simulink model "P_decouple_cascade_rov"  (Simulink 6.0)
settings: Solver=ode45  StartTime=0.0  StopTime=650  RelTol=1e-3
undefined symbols (not defined in the file): B, DQ, DQL, I, m, M, Ma, MaL, MaU, rg, sigbuilder_block, T, W, xb, xg, Xudot, yb, yg, Yvdot, zb, zg, Zwdot
libraries: simulink_extras x27, simulink x20
(part 1 of 5)
settings Model: LastModifiedBy=c chin

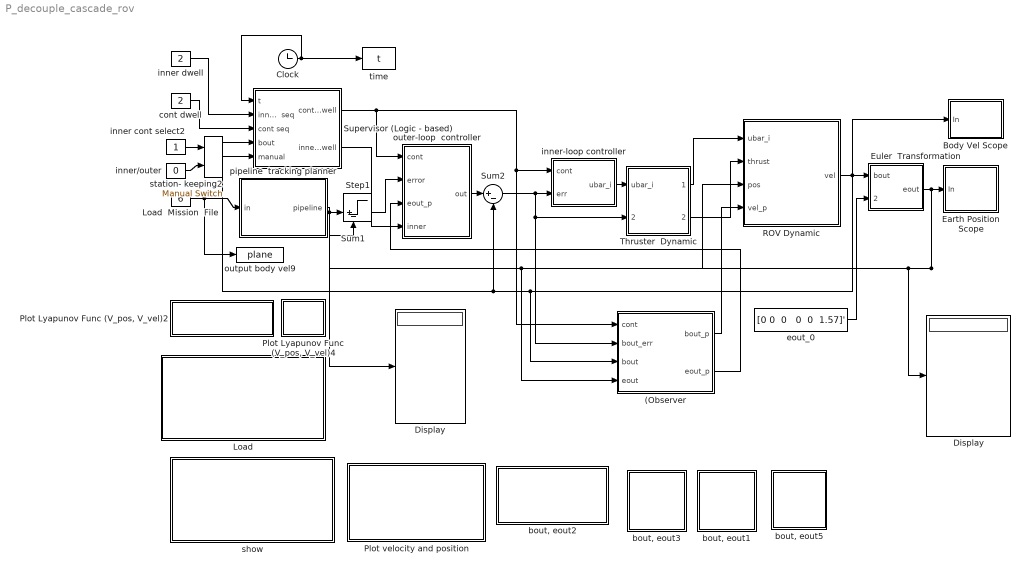
== system P_decouple_cascade_rov ==
  " Load  " : Subsystem  AncestorBlock=|
      | rov_design_analysis/ROV Controller
      | Design
      | Applications/ Load RRCROV2 parameters
      settings: OpenFcn=|
      | clc
      | cd c:\Matlab7\toolbox\rov_design_analysis\\mat_file ;
      | load rrcrovf;
      mask Display: disp('Double-click \n to \n Load the\n RRCROV\n parameters')
  " ROV Dynamic   " : Subsystem
      mask Display:
      | disp('ROV')
      | image(imread('/rov_design_analysis/fig/ROVRRC2.jpg'));
      | color('white');port_label('input',1,'ubar_i')
      | color('white');port_label('input',2,'thrust')
      | color('white');port_label('input',3,'MCD_select')
      | color('white');port_label('input',4,'eout')
      | color('white');port_label('input',5,'bout_p')
      | 
      | color('white');port_label('output',1,'vel')
      | color('white');port_label('output',2,'boutdot')
  " inner dwell" : Constant  Value=2
  " station- keeping2" : simulink/Signal Routing/Manual Switch  sw=1  action=0
  (Observer : Subsystem
      mask Display: disp('Observer')
  Body Vel Scope : Subsystem  AncestorBlock=|
      | rov_design_analysis/ROV Controller
      | Design
      | Applications/1. Heading autopilot/Earth Position
      | Scope
      mask Display: disp('Body\nVelocity\nScope')
  Clock : Clock
      settings: Decimation=10
  Display : Display
  "Display " : Display
  "Earth Position Scope " : Subsystem  AncestorBlock=|
      | rov_design_analysis/ROV Controller
      | Design
      | Applications/1. Heading autopilot/Earth Position
      | Scope
      mask Display: disp('Earth\nPosition\nScope')
  Euler  Transformation : Subsystem  AncestorBlock=rov_design_analysis/Scope Utilities/Euler Transformation
      mask Display: disp('Navigation \n Sensor')
  Load  Mission  File : Constant  Value=6
  "Plot Lyapunov Func (V_pos, V_vel)2" : Subsystem  AncestorBlock=|
      | rov_design_analysis/ROV Controller
      | Design
      | Applications/Plot velocity and position
      settings: OpenFcn=|
      | clc
      | close all
      mask Display: disp('Close All Figure')
  "Plot Lyapunov Func (V_pos, V_vel)4" : Subsystem  AncestorBlock=|
      | rov_design_analysis/ROV Controller
      | Design
      | Applications/Plot velocity and position
      settings: OpenFcn=|
      | clc
      | clear
      mask Display: disp('Clear')
  Plot velocity and position : Subsystem  AncestorBlock=|
      | rov_design_analysis/ROV Controller
      | Design
      | Applications/Plot velocity and position
      settings: OpenFcn=|
      | clc
      | cd c:\Matlab7\toolbox\rov_design_analysis\\m_file ;
      | run nonlin_resp6
      mask Display: disp('Double-click \n to \n Plot Velocity \n and \n Position')
  Sum1 : Sum  Inputs=|+-  OutDataTypeMode=double  SaturateOnIntegerOverflow=on
  Sum2 : Sum  Inputs=|+-  OutDataTypeMode=double  SaturateOnIntegerOverflow=on
  Supervisor (Logic - based) : Subsystem
      mask Display: disp('Supervisor \n (Logic-based)')
  Thruster  Dynamic : Subsystem
      mask Display: disp('Thruster \n Dynamic')
  "bout, eout1" : Subsystem  AncestorBlock=|
      | rov_design_analysis/ROV Controller
      | Design
      | Applications/Plot velocity and position
      settings: OpenFcn=|
      | clc
      | cd c:\Matlab7\toolbox\rov_design_analysis\\m_file ;
      | figure
      | plot(eout(:,1),-eout(:,3))
      | xlabel('x')
      | ylabel('z')
      mask Display: disp('Plot \n XZ ')
  "bout, eout2" : Subsystem  AncestorBlock=|
      | rov_design_analysis/ROV Controller
      | Design
      | Applications/Plot velocity and position
      settings: OpenFcn=|
      | clc
      | cd c:\Matlab7\toolbox\rov_design_analysis\\m_file ;
      | figure
      | plot3(eout(:,1), eout(:,2),-eout(:,3))
      | xlabel('x')
      | ylabel('y')
      | zlabel('z')
      | grid on
      mask Display: disp('Plot \n 3D Response')
  "bout, eout3" : Subsystem  AncestorBlock=|
      | rov_design_analysis/ROV Controller
      | Design
      | Applications/Plot velocity and position
      settings: OpenFcn=|
      | clc
      | cd c:\Matlab7\toolbox\rov_design_analysis\\m_file ;
      | figure
      | plot(eout(:,1), eout(:,2))
      | xlabel('x')
      | ylabel('y')
      mask Display: disp('Plot \n XY ')
  "bout, eout5" : Subsystem  AncestorBlock=|
      | rov_design_analysis/ROV Controller
      | Design
      | Applications/Plot velocity and position
      settings: OpenFcn=|
      | clc
      | cd c:\Matlab7\toolbox\rov_design_analysis\\m_file ;
      | figure
      | box off
      | subplot(4,1,1)
      | plot(inner.time,inner.signals.values)
      | xlabel('time (sec)')
      | ylabel('Inner controller type')
      | subplot(4,1,2)
      | plot(outer.time,outer.signals.values)
      | xlabel('time (sec)')
      | ylabel('Outer controller type')
      | subplot(4,1,3)
      | plot(plane.time,plane.signals.values)
      | xlabel('time (sec)')
      | ylabel('Input sequence')
      | 
      | subplot(4,1,4)
      | plot(inner_only.time,inner_only.signals.values)
      | xlabel('time (sec)')
      | ylabel('Inner/Outer loop')
      mask Display: disp('Plot \n switching \n signal ')
  cont dwell : Constant  Value=2
  eout_0 : Constant  Value="[0 0  0   0  0  1.57]'"  OutDataTypeMode=double
  inner cont select2 : Constant
  inner-loop controller : Subsystem  Description=f(x)  AncestorBlock=|
      | rov_design_analysis/ROV Controller
      | Design
      | Applications/1. Heading autopilot/controller
      mask Display: disp('Inner Loop \n Controller')
  "inner/outer  " : Constant  Value=0
  outer-loop  controller : Subsystem  Description=f(x)  AncestorBlock=|
      | rov_design_analysis/ROV Controller
      | Design
      | Applications/1. Heading autopilot/controller
      mask Display: disp('Outer Loop \n Controller')
  output body vel9 : ToWorkspace  VariableName=plane  SampleTime=1  SaveFormat=Structure With Time
  "pipeline  tracking planner  " : Subsystem  AncestorBlock=|
      | rov_design_analysis/ROV Controller
      | Design
      | Applications/1. Heading autopilot/pipe tracking
      | profile
      | (Auto)
      mask Display: disp('Pipeline Tracking \n Planner')
  show : Subsystem  AncestorBlock=|
      | rov_design_analysis/ROV Controller
      | Design
      | Applications/ Load RRCROV2 parameters
      settings: OpenFcn=|
      | clc
      | cd  c:\Matlab7\toolbox\rov_design_analysis\hybrid ;
      | open rrcrov2_para
      mask Display: disp('Double-click \n to \n SHOW\n RRCROV\n parameters')
  time : ToWorkspace  VariableName=t  SampleTime=1  SaveFormat=Array
  Step1 : Step  IOType=siggen  SampleTime=0
  wires:
  " ROV Dynamic   "/1(vel) -> Euler  Transformation/1(bout), (Observer/3(bout), Sum2/2, Supervisor (Logic - based)/4(bout), Body Vel Scope/1(In)
  Euler  Transformation/1(eout) -> "Earth Position Scope "/1(In), (Observer/4(eout), Sum1/2, " ROV Dynamic   "/3("pos "), "Display "/1
  Clock/1 -> time/1, Supervisor (Logic - based)/1(t)
  Thruster  Dynamic/2(thruster_out) -> " ROV Dynamic   "/2("thrust ")
  Sum2/1 -> Thruster  Dynamic/2(bout_err), (Observer/2(bout_err), inner-loop controller/2(err)
  Thruster  Dynamic/1(cont_out) -> " ROV Dynamic   "/1(ubar_i)
  inner-loop controller/1(ubar_i) -> Thruster  Dynamic/1(ubar_i)
  (Observer/2(eout_p) -> outer-loop  controller/3(eout_p)
  (Observer/1(bout_p) -> " ROV Dynamic   "/4(vel_p)
  "pipeline  tracking planner  "/1(pipeline) -> Sum1/1, Display/1
  Supervisor (Logic - based)/1(cont dwell) -> inner-loop controller/1(cont), (Observer/1(cont), outer-loop  controller/1(cont)
  outer-loop  controller/1(out) -> Sum2/1
  Supervisor (Logic - based)/2(inner  dwell) -> outer-loop  controller/4(inner)
  " inner dwell"/1 -> Supervisor (Logic - based)/2(inner  seq)
  cont dwell/1 -> Supervisor (Logic - based)/3(cont seq)
  eout_0/1 -> Euler  Transformation/2(eout_0)
  Load  Mission  File/1 -> output body vel9/1, "pipeline  tracking planner  "/1(in)
  inner cont select2/1 -> " station- keeping2"/1
  "inner/outer  "/1 -> " station- keeping2"/2
  " station- keeping2"/1 -> Supervisor (Logic - based)/5(manual)
  Sum1/1 -> outer-loop  controller/2(error)

== system P_decouple_cascade_rov/ Load   ==

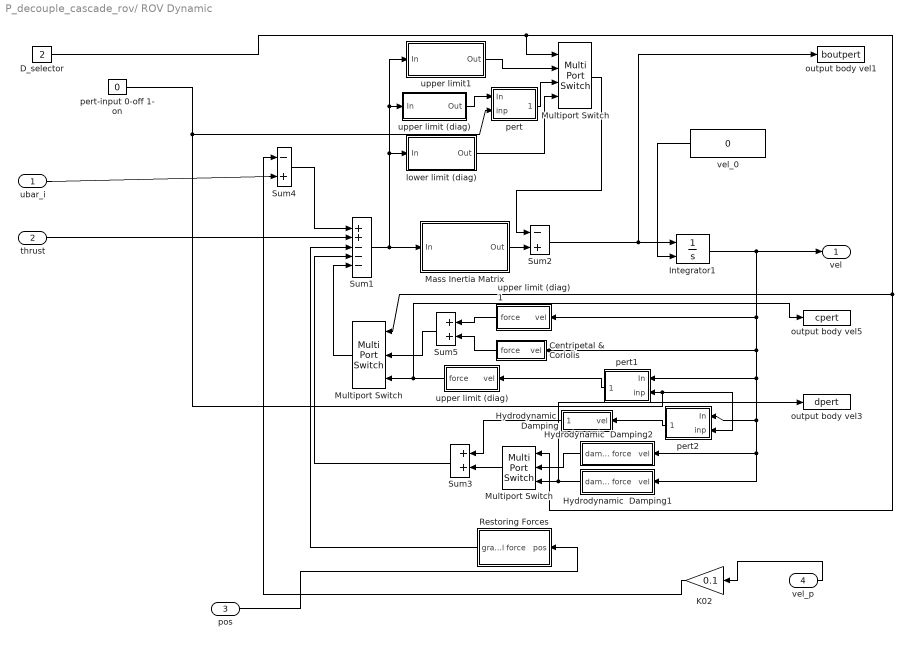
== system P_decouple_cascade_rov/ ROV Dynamic    ==
  ubar_i : Inport  Port=1  LatchInput=off
  "thrust " : Inport  Port=2  LatchInput=off
  "pos " : Inport  Port=3  LatchInput=off
  vel_p : Inport  Port=4  LatchInput=off
  Centripetal & Coriolis : Subsystem  Orientation=left  AncestorBlock=rov_design_analysis/ROV Models/1. Six DOF RRC ROV II/Centripetal & Coriolis
      mask Display: disp('C')
  D_selector : Constant  Value=2
  Hydrodynamic  Damping : Subsystem  Orientation=left
      mask Display: disp('D')
  Hydrodynamic  Damping1 : Subsystem  Orientation=left
      mask Display: disp('perturb \nDamping')
  Hydrodynamic  Damping2 : Subsystem  Orientation=left
      mask Display: disp('Zero Perturb')
  Integrator1 : Integrator  InitialConditionSource=external
  K02 : Gain  Orientation=left  Gain=0.1  SaturateOnIntegerOverflow=on
  Mass Inertia Matrix : Subsystem
      mask Display: disp('inv(MRB+MA)')
  Multiport Switch : MultiPortSwitch  Inputs=3
  "Multiport Switch  " : MultiPortSwitch  Orientation=left  Inputs=2
  "Multiport Switch    " : MultiPortSwitch  Orientation=left  Inputs=2
  Restoring Forces : Subsystem  Orientation=left
      mask Display: disp('Restoring\nForce')
  Sum1 : Sum  Inputs=++---  SaturateOnIntegerOverflow=on  InputSameDT=on
  Sum2 : Sum  Inputs=-+  SaturateOnIntegerOverflow=on  InputSameDT=on
  Sum3 : Sum  Orientation=left  SaturateOnIntegerOverflow=on  InputSameDT=on
  Sum4 : Sum  Inputs=|-+  SaturateOnIntegerOverflow=on  InputSameDT=on
  Sum5 : Sum  Orientation=left  SaturateOnIntegerOverflow=on  InputSameDT=on
  lower limit (diag) : Subsystem
      mask Display: disp('Perturb MA')
  output body vel1 : ToWorkspace  VariableName=boutpert  SampleTime=1  SaveFormat=Array
  output body vel3 : ToWorkspace  VariableName=dpert  SampleTime=1  SaveFormat=Array
  output body vel5 : ToWorkspace  VariableName=cpert  SampleTime=1  SaveFormat=Array
  pert : Subsystem
  pert-input 0-off 1- on : Constant  Value=0
  pert1 : Subsystem  Orientation=left
  pert2 : Subsystem  Orientation=left
  upper limit (diag) : Subsystem
      mask Display: disp('Perturb MA')
  "upper limit (diag)   " : Subsystem  Orientation=left
      mask Display: disp('Perturb CA')
  upper limit (diag)   1 : Subsystem  Orientation=left
      mask Display: disp('CA')
  upper limit1 : Subsystem
      mask Display: disp('Zero Perturb')
  vel_0 : Constant  Orientation=left  Value=0  OutDataTypeMode=double
  vel : Outport
  wires:
  Restoring Forces/1(gravitational force) -> Sum1/3
  "thrust "/1 -> Sum1/2
  Sum1/1 -> Mass Inertia Matrix/1(In), upper limit1/1(In), upper limit (diag)/1(In), lower limit (diag)/1(In)
  "Multiport Switch  "/1 -> Sum1/5
  "pos "/1 -> Restoring Forces/1(pos)
  Mass Inertia Matrix/1(Out) -> Sum2/2
  upper limit1/1(Out) -> Multiport Switch/2
  lower limit (diag)/1(Out) -> Multiport Switch/4
  Multiport Switch/1 -> Sum2/1
  "upper limit (diag)   "/1(force) -> "Multiport Switch  "/3, output body vel5/1
  Sum5/1 -> "Multiport Switch  "/2
  Hydrodynamic  Damping1/1(damping force) -> "Multiport Switch    "/3, output body vel3/1
  Hydrodynamic  Damping2/1(damping force) -> "Multiport Switch    "/2
  Sum3/1 -> Sum1/4
  "Multiport Switch    "/1 -> Sum3/2
  Hydrodynamic  Damping/1(damping force) -> Sum3/1
  upper limit (diag)   1/1(force) -> Sum5/1
  Centripetal & Coriolis/1(force) -> Sum5/2
  Sum2/1 -> output body vel1/1, Integrator1/1
  Integrator1/1 -> vel/1, upper limit (diag)   1/1(vel), Centripetal & Coriolis/1(vel), Hydrodynamic  Damping1/1(vel), Hydrodynamic  Damping2/1(vel), pert2/1(In), pert1/1(In)
  vel_0/1 -> Integrator1/2
  K02/1 -> Sum4/1
  ubar_i/1 -> Sum4/2
  Sum4/1 -> Sum1/1
  vel_p/1 -> K02/1
  pert2/1(on/off) -> Hydrodynamic  Damping/1(vel)
  pert1/1(on/off) -> "upper limit (diag)   "/1(vel)
  upper limit (diag)/1(Out) -> pert/1(In)
  pert/1(on/off) -> Multiport Switch/3
  pert-input 0-off 1- on/1 -> pert/2(inp), pert1/2(inp), pert2/2(inp)
  D_selector/1 -> Multiport Switch/1, "Multiport Switch  "/1, "Multiport Switch    "/1

== system P_decouple_cascade_rov/(Observer ==
  cont : Inport  Port=1  LatchInput=off
  bout_err : Inport  Port=2  LatchInput=off
  bout : Inport  Port=3  LatchInput=off
  eout : Inport  Port=4  LatchInput=off
  " Six DOF RRC ROV   1" : Subsystem
      mask Display:
      | disp('ROV')
      | image(imread('/rov_design_analysis/fig/ROVRRC2.jpg'));
      | color('white');port_label('input',1,'ubar_i')
      | color('white');port_label('input',2,'thrust')
      | color('white');port_label('input',3,'MCD_select')
      | color('white');port_label('input',4,'pos')
      | color('white');port_label('output',1,'vel')
      | color('white');port_label('output',2,'Inv_MC')
  Euler  Transformation1 : Subsystem  AncestorBlock=rov_design_analysis/Scope Utilities/Euler Transformation
  MCD_selector : Constant  Value=2
  Sum1 : Sum  Inputs=-+  SaturateOnIntegerOverflow=on  InputSameDT=on
  Sum2 : Sum  Inputs=-+  SaturateOnIntegerOverflow=on  InputSameDT=on
  Thruster  Dynamic : Subsystem
  eout_hat_0 : Constant  Orientation=left  Value=0  OutDataTypeMode=double
  inner-loop controller1 : Subsystem  Description=f(x)  AncestorBlock=|
      | rov_design_analysis/ROV Controller
      | Design
      | Applications/1. Heading autopilot/controller
  output body vel2 : ToWorkspace  VariableName=boutupert  SampleTime=1  SaveFormat=Array
  output body vel4 : ToWorkspace  VariableName=eoutupert  SampleTime=1  SaveFormat=Array
  bout_p : Outport
  eout_p : Outport  Port=2
  wires:
  " Six DOF RRC ROV   1"/1(vel) -> Euler  Transformation1/1(vel), Sum2/1, output body vel2/1
  MCD_selector/1 -> " Six DOF RRC ROV   1"/3(MCD_select), inner-loop controller1/3(M_select)
  bout_err/1 -> Thruster  Dynamic/2(bout_err), inner-loop controller1/2(err)
  Euler  Transformation1/1(eout_hat) -> " Six DOF RRC ROV   1"/4("pos "), Sum1/1, output body vel4/1
  eout_hat_0/1 -> Euler  Transformation1/2(eta_0)
  bout/1 -> Sum2/2
  eout/1 -> Sum1/2
  Sum2/1 -> bout_p/1
  Sum1/1 -> eout_p/1
  Thruster  Dynamic/1(cont_out) -> " Six DOF RRC ROV   1"/1(ubar_i)
  inner-loop controller1/1(ubar_i) -> Thruster  Dynamic/1(ubar_i)
  Thruster  Dynamic/2(thruster_out) -> " Six DOF RRC ROV   1"/2("thrust ")
  cont/1 -> inner-loop controller1/1(cont)

== system P_decouple_cascade_rov/Body Vel Scope ==
  In : Inport  Port=1  LatchInput=off
  Demux : Demux  Outputs=6
  output body vel4 : ToWorkspace  VariableName=bout  SampleTime=1  SaveFormat=Array
  phi : Scope
      settings: TickLabels=on  YMin=-0.125  YMax=0.2  DataFormat=Array
  theta : Scope
      settings: TickLabels=on  TimeRange=200  YMin=-0.05  YMax=0.15  DataFormat=Array
  x : Scope
      settings: TickLabels=on  TimeRange=50  YMin=-0.025  YMax=0.375  DataFormat=Array
  y : Scope
      settings: TickLabels=on  YMin=-0.02  YMax=0.1  DataFormat=Array
  yaw : Scope
      settings: TickLabels=on  TimeRange=200  YMin=-0.05  YMax=0.15  SaveName=ScopeData2  DataFormat=Array
  z : Scope
      settings: TickLabels=on  TimeRange=50  YMin=-0.0025  YMax=0.0375  DataFormat=Array
  wires:
  Demux/5 -> theta/1
  In/1 -> Demux/1, output body vel4/1
  Demux/3 -> z/1
  Demux/4 -> phi/1
  Demux/2 -> y/1
  Demux/1 -> x/1
  Demux/6 -> yaw/1

== system P_decouple_cascade_rov/Earth Position Scope  ==
  In : Inport  Port=1  LatchInput=off
  Demux : Demux  Outputs=6
  XY Graph : simulink/Sinks/XY Graph  xmin=-50  xmax=50  ymin=-50  ymax=50  st=-1
  output body vel5 : ToWorkspace  VariableName=eout  SampleTime=1  SaveFormat=Array
  phi : Scope
      settings: TickLabels=on  YMin=-0.125  YMax=0.2  DataFormat=Array
  theta : Scope
      settings: TickLabels=on  TimeRange=200  YMin=-0.05  YMax=0.15  DataFormat=Array
  x : Scope
      settings: TickLabels=on  TimeRange=50  YMin=-0.025  YMax=0.375  DataFormat=Array
  y : Scope
      settings: TickLabels=on  YMin=-0.02  YMax=0.1  DataFormat=Array
  yaw : Scope
      settings: TickLabels=on  TimeRange=200  YMin=-0.05  YMax=0.15  SaveName=ScopeData2  DataFormat=Array
  z : Scope
      settings: TickLabels=on  TimeRange=50  YMin=-0.0025  YMax=0.0375  DataFormat=Array
  wires:
  Demux/5 -> theta/1
  In/1 -> Demux/1, output body vel5/1
  Demux/3 -> z/1
  Demux/4 -> phi/1
  Demux/2 -> y/1, XY Graph/2
  Demux/1 -> x/1, XY Graph/1
  Demux/6 -> yaw/1

== system P_decouple_cascade_rov/Euler  Transformation ==
  bout : Inport  Port=1  LatchInput=off
  eout_0 : Inport  Port=2  LatchInput=off
  Demux : Demux  Outputs=2
  Demux1 : Demux  Outputs=2
  Intregrator2 : Integrator  InitialConditionSource=external
  Mux1 : Mux  Inputs=2
  Terminator : Terminator
  Transformation matrix R : Subsystem
      mask Display: disp('Transformation R')
  Transformation matrix T : Subsystem
      mask Display: disp('Transformation T')
  output body vel1 : ToWorkspace  VariableName=eoutpert  SampleTime=1  SaveFormat=Array
  eout : Outport  InitialOutput=0
  wires:
  Mux1/1 -> Intregrator2/1
  Intregrator2/1 -> Demux1/1, eout/1, output body vel1/1
  Demux/2 -> Transformation matrix R/1(angular body  velocity)
  Demux/1 -> Transformation matrix T/1(translational body velocity)
  bout/1 -> Demux/1
  Demux1/2 -> Transformation matrix T/2(angular position), Transformation matrix R/2(angular position)
  Transformation matrix R/1(angular earth velocity) -> Mux1/2
  Transformation matrix T/1(translational earth velocity) -> Mux1/1
  Demux1/1 -> Terminator/1
  eout_0/1 -> Intregrator2/2

== system P_decouple_cascade_rov/Plot Lyapunov Func (V_pos, V_vel)2 ==

== system P_decouple_cascade_rov/Plot Lyapunov Func (V_pos, V_vel)4 ==

== system P_decouple_cascade_rov/Plot velocity and position ==

== system P_decouple_cascade_rov/Supervisor (Logic - based) ==
  t : Inport  Port=1  LatchInput=off
  inner  seq : Inport  Port=2  LatchInput=off
  cont seq : Inport  Port=3  LatchInput=off
  bout : Inport  Port=4  LatchInput=off
  manual : Inport  Port=5  LatchInput=off
  150-300 : Relay  OnSwitchValue=150  OffSwitchValue=0  OnOutputValue=0  OffOutputValue=1
  Constant1 : Constant
  Constant8 : Constant
  Gain : Gain  Gain=0.5
  Mass Inertia Matrix1 : Subsystem
      mask Display: disp('MRB+MA')
  Math Function1 : Math  Operator=square  SaturateOnIntegerOverflow=on
  Subsystem : Subsystem
  Switching sequence : Subsystem  AncestorBlock=rov_design_analysis/Scope Utilities/Switching sequence
      mask Display: disp('Dwell \n Sequence')
  Switching sequence1 : Subsystem  AncestorBlock=rov_design_analysis/Scope Utilities/Switching sequence
      mask Display: disp('Dwell \n Sequence')
  "cont dwell switch  " : MultiPortSwitch  Inputs=2
  inner dwell Switch : MultiPortSwitch  Inputs=3
  output body vel6 : ToWorkspace  VariableName=outer  SampleTime=1  SaveFormat=Structure With Time
  output body vel8 : ToWorkspace  VariableName=inner_only  SampleTime=1  SaveFormat=Structure With Time
  cont dwell : Outport
  inner  dwell : Outport  Port=2
  wires:
  inner  seq/1 -> inner dwell Switch/1
  150-300/1 -> inner dwell Switch/2  "1"
  Constant8/1 -> inner dwell Switch/3  "2"
  inner dwell Switch/1 -> Subsystem/1(In)
  cont seq/1 -> "cont dwell switch  "/1
  "cont dwell switch  "/1 -> cont dwell/1, output body vel6/1
  t/1 -> 150-300/1
  Switching sequence1/1(" ") -> "cont dwell switch  "/2
  Constant1/1 -> "cont dwell switch  "/3
  Switching sequence/1(" ") -> inner dwell Switch/4  "3"
  Subsystem/1(inner dwell) -> inner  dwell/1, output body vel8/1
  manual/1 -> Subsystem/3(manual)
  bout/1 -> Math Function1/1
  Math Function1/1 -> Mass Inertia Matrix1/1(In)
  Mass Inertia Matrix1/1(Out) -> Gain/1
  Gain/1 -> Subsystem/2(V)

== system P_decouple_cascade_rov/Thruster  Dynamic ==
  ubar_i : Inport  Port=1  LatchInput=off
  bout_err : Inport  Port=2  LatchInput=off
  Sum2 : Sum  Inputs=|++  OutDataTypeMode=double  SaturateOnIntegerOverflow=on
  Thruster configuration1 : Subsystem  AncestorBlock=|
      | rov_design_analysis/ROV Controller
      | Design
      | Applications/1. Heading autopilot/Thruster
      | configuration
      mask Display: disp('T')
  Thruster configuration4 : Subsystem  AncestorBlock=|
      | rov_design_analysis/ROV Controller
      | Design
      | Applications/1. Heading autopilot/Thruster
      | configuration
      mask Display: disp('T')
  output earth pos1 : ToWorkspace  VariableName=thrustdc  SampleTime=1  SaveFormat=Array
  output earth pos2 : ToWorkspace  VariableName=thrustd  SampleTime=1  SaveFormat=Array
  output earth pos3 : ToWorkspace  VariableName=thrust  SampleTime=1  SaveFormat=Array
  thruster  dynamic     1 : Subsystem
  cont_out : Outport
  thruster_out : Outport  Port=2
  wires:
  Thruster configuration1/1(output force) -> thruster_out/1
  Thruster configuration4/1(output force) -> cont_out/1
  thruster  dynamic     1/1(T) -> Thruster configuration1/1(input velocity), Sum2/2, output earth pos3/1
  bout_err/1 -> thruster  dynamic     1/1(volt)
  ubar_i/1 -> Thruster configuration4/1(input velocity), Sum2/1, output earth pos1/1
  Sum2/1 -> output earth pos2/1

== system P_decouple_cascade_rov/bout, eout1 ==

== system P_decouple_cascade_rov/bout, eout2 ==

== system P_decouple_cascade_rov/bout, eout3 ==

== system P_decouple_cascade_rov/bout, eout5 ==

== system P_decouple_cascade_rov/inner-loop controller ==
  cont : Inport  Port=1  LatchInput=off
  err : Inport  Port=2  LatchInput=off
  MCD_selector : Constant  Value=2
  Multiport Switch : MultiPortSwitch
  "inner -PI-decouple " : Subsystem
  inner -backstepping : Subsystem
  inner-P : Subsystem
  inner-sliding : Subsystem
  output body vel7 : ToWorkspace  VariableName=inner  SampleTime=1  SaveFormat=Structure With Time
  ubar_i : Outport
  wires:
  Multiport Switch/1 -> ubar_i/1
  cont/1 -> Multiport Switch/1, output body vel7/1
  "inner -PI-decouple "/1(" ") -> Multiport Switch/2
  inner-P/1(" ") -> Multiport Switch/3
  err/1 -> inner-P/1(P), inner-sliding/1(sliding), inner -backstepping/1(err), "inner -PI-decouple "/1(err)
  inner -backstepping/1(" ") -> Multiport Switch/4
  inner-sliding/1(" ") -> Multiport Switch/5
  MCD_selector/1 -> inner -backstepping/2(M_select)

== system P_decouple_cascade_rov/outer-loop  controller ==
  cont : Inport  Port=1  LatchInput=off
  error : Inport  Port=2  LatchInput=off
  eout_p : Inport  Port=3  LatchInput=off
  inner : Inport  Port=4  LatchInput=off
  K01 : Gain  Gain=0.1  SaturateOnIntegerOverflow=on
  Multiport Switch : MultiPortSwitch
  P : Subsystem
  "PI sine +nonlinear " : Subsystem
  Product1 : Product  RndMeth=Zero
  Sum3 : Sum  Inputs=|++  SaturateOnIntegerOverflow=on  InputSameDT=on
  Sum4 : Sum  Inputs=|-+  SaturateOnIntegerOverflow=on  InputSameDT=on
  bout input : Constant  Value="[ 0 0  0  0  0 0]'"
  "outer-P decouple " : Subsystem
  outer-sliding decouple : Subsystem
  out : Outport
  wires:
  Multiport Switch/1 -> Product1/2
  cont/1 -> Multiport Switch/1
  bout input/1 -> Sum3/1, outer-sliding decouple/2(vel_d), "outer-P decouple "/2(vel_d)
  "outer-P decouple "/1(" ") -> Multiport Switch/2
  P/1(" ") -> Multiport Switch/3
  error/1 -> Sum4/2
  Sum4/1 -> "outer-P decouple "/1(err), P/1(err), outer-sliding decouple/1(err), "PI sine +nonlinear "/1(err)
  K01/1 -> Sum4/1
  eout_p/1 -> K01/1
  inner/1 -> Product1/1
  Product1/1 -> Sum3/2
  Sum3/1 -> out/1
  outer-sliding decouple/1(" ") -> Multiport Switch/4
  "PI sine +nonlinear "/1(" ") -> Multiport Switch/5

== system P_decouple_cascade_rov/pipeline  tracking planner   ==
  in : Inport  Port=1  LatchInput=off
  decoupled input : Subsystem
  pipeline : Outport
  wires:
  in/1 -> decoupled input/1(In1)
  decoupled input/1(Out1) -> pipeline/1

== system P_decouple_cascade_rov/show ==

== system P_decouple_cascade_rov/ ROV Dynamic   /Centripetal & Coriolis ==
  vel : Inport  Orientation=up  Port=1  LatchInput=off
  Demux : Demux  Orientation=up  Outputs=2
  Mux : Mux  Inputs=2
  Product{1..5} (5 alike) : Product  SaturateOnIntegerOverflow=on  RndMeth=Zero  InputSameDT=on
  Rg : Constant  Value=rg
  Sum : Sum  SaturateOnIntegerOverflow=on  InputSameDT=on
  Sum1 : Sum  SaturateOnIntegerOverflow=on  InputSameDT=on
  inertia(3x3) : Gain  Gain=I*eye(3)+[Xudot 0 0;0 Yvdot 0;0 0 Zwdot]  Multiplication=Matrix(K*u)  SaturateOnIntegerOverflow=on
  "mass(3x3) " : Gain  Gain=m*eye(3)+[Xudot 0 0;0 Yvdot 0;0 0 Zwdot]  Multiplication=Matrix(K*u)  SaturateOnIntegerOverflow=on
  "mass(3x3)   " : Gain  Gain=m*eye(3)+[Xudot 0 0;0 Yvdot 0;0 0 Zwdot]  Multiplication=Matrix(K*u)  SaturateOnIntegerOverflow=on
  force : Outport  InitialOutput=0
  wires:
  Product1/1 -> Sum/2
  "mass(3x3)   "/1 -> Product2/1
  Product2/1 -> Sum/1
  Rg/1 -> Product3/2, "mass(3x3)   "/1
  Product3/1 -> Product4/2
  Product4/1 -> Sum1/1
  Product5/1 -> Product2/2, Sum1/2
  Sum1/1 -> "mass(3x3) "/1
  Demux/2 -> Product5/1, Product3/1, Product4/1, Product1/1, inertia(3x3)/1
  Demux/1 -> Product5/2
  vel/1 -> Demux/1
  inertia(3x3)/1 -> Product1/2
  "mass(3x3) "/1 -> Mux/1
  Sum/1 -> Mux/2
  Mux/1 -> force/1

== system P_decouple_cascade_rov/ ROV Dynamic   /Hydrodynamic  Damping ==
  vel : Inport  Port=1  LatchInput=off
  D linear : Gain  Gain=-diag(DQL)  SaturateOnIntegerOverflow=on
  damping force : Outport  InitialOutput=0
  wires:
  vel/1 -> D linear/1
  D linear/1 -> damping force/1

== system P_decouple_cascade_rov/ ROV Dynamic   /Hydrodynamic  Damping1 ==
  vel : Inport  Port=1  LatchInput=off
  D quadratic : Gain  Gain=-diag(DQ)  SaturateOnIntegerOverflow=on
  Product : Product  SaturateOnIntegerOverflow=on  RndMeth=Zero  InputSameDT=on
  |u| : Abs  SaturateOnIntegerOverflow=on
  damping force : Outport  InitialOutput=0
  wires:
  Product/1 -> D quadratic/1
  vel/1 -> Product/1, |u|/1
  |u|/1 -> Product/2
  D quadratic/1 -> damping force/1

== system P_decouple_cascade_rov/ ROV Dynamic   /Hydrodynamic  Damping2 ==
  vel : Inport  Port=1  LatchInput=off
  D quadratic : Gain  Gain=0  SaturateOnIntegerOverflow=on
  damping force : Outport  InitialOutput=0
  wires:
  D quadratic/1 -> damping force/1
  vel/1 -> D quadratic/1

== system P_decouple_cascade_rov/ ROV Dynamic   /Mass Inertia Matrix ==
  In : Inport  Port=1  LatchInput=off
  inverse M : Gain  Gain=inv(M-Ma)  Multiplication=Matrix(K*u)  SaturateOnIntegerOverflow=on
  Out : Outport
  wires:
  inverse M/1 -> Out/1
  In/1 -> inverse M/1

== system P_decouple_cascade_rov/ ROV Dynamic   /Restoring Forces ==
  pos : Inport  Port=1  LatchInput=off
  (xg.W-xb.B)cY.cX : Fcn  Expr=(xg*W - xb*B)*cos(u[2])*cos(u[1])
  (zg.W - zb.B)cY.sX : Fcn  Expr=((zg * W - zb * B) * cos(u[2])) * sin(u[1])
  (zg.W - zb.B)sY : Fcn  Expr=(zg*W - zb*B)*sin(u[2])
  -(xg.W-xb.B)cY.sX : Fcn  Expr=-(xg*W - xb*B)*cos(u[2])*sin(u[1])
  -(yg.W-yb.B)cY.cX : Fcn  Expr=-(yg*W - yb*B)*cos(u[2])*cos(u[1])
  -(yg.W-yb.B)sY : Fcn  Expr=-(yg*W - yb*B)*sin(u[2])
  -cY.cX : Fcn  Expr=-cos(u[2])*cos(u[1])
  -cY.sX : Fcn  Expr=-cos(u[2])*sin(u[1])
  Demux : Demux  Outputs=2
  Gain : Gain  Gain=W-B  SaturateOnIntegerOverflow=on
  Mux : Mux  Inputs=3
  Mux1 : Mux
  Sum : Sum  SaturateOnIntegerOverflow=on  InputSameDT=on
  Sum1 : Sum  SaturateOnIntegerOverflow=on  InputSameDT=on
  Sum2 : Sum  SaturateOnIntegerOverflow=on  InputSameDT=on
  Terminator : Terminator
  sY : Fcn  Expr=sin(u[2])
  gravitational force : Outport  InitialOutput=0
  wires:
  Sum2/1 -> Mux1/4
  -(yg.W-yb.B)sY/1 -> Sum2/1
  -(xg.W-xb.B)cY.sX/1 -> Sum2/2
  Sum1/1 -> Mux1/3
  (xg.W-xb.B)cY.cX/1 -> Sum1/1
  (zg.W - zb.B)sY/1 -> Sum1/2
  Sum/1 -> Mux1/2
  (zg.W - zb.B)cY.sX/1 -> Sum/1
  -(yg.W-yb.B)cY.cX/1 -> Sum/2
  Gain/1 -> Mux1/1
  Mux/1 -> Gain/1
  -cY.cX/1 -> Mux/3
  -cY.sX/1 -> Mux/2
  sY/1 -> Mux/1
  Mux1/1 -> gravitational force/1
  Demux/2 -> -(xg.W-xb.B)cY.sX/1, -(yg.W-yb.B)sY/1, (zg.W - zb.B)sY/1, (xg.W-xb.B)cY.cX/1, -(yg.W-yb.B)cY.cX/1, (zg.W - zb.B)cY.sX/1, sY/1, -cY.sX/1, -cY.cX/1
  Demux/1 -> Terminator/1
  pos/1 -> Demux/1

== system P_decouple_cascade_rov/ ROV Dynamic   /lower limit (diag) ==
  In : Inport  Port=1  LatchInput=off
  inverse M : Gain  Gain=-diag([21.1403-21.0981 51.7012-51.0026 92.451-91.837 3.6191-3.576 2.6427-2.7687 2.3033-2.3493])  Multiplication=Matrix(K*u)  SaturateOnIntegerOverflow=on
  Out : Outport
  wires:
  inverse M/1 -> Out/1
  In/1 -> inverse M/1

== system P_decouple_cascade_rov/ ROV Dynamic   /pert ==
  In : Inport  Port=1  LatchInput=off
  inp : Inport  Port=2  LatchInput=off
  D linear3 : Gain  Gain=2  SaturateOnIntegerOverflow=on
  Product : Product  RndMeth=Zero
  Sine Wave-pert : Sin  Amplitude=0.1  SampleTime=0
  Sum6 : Sum  Inputs=|++  SaturateOnIntegerOverflow=on  InputSameDT=on
  on/off : Outport
  wires:
  D linear3/1 -> Sum6/1
  Sine Wave-pert/1 -> Product/1
  Product/1 -> Sum6/2
  inp/1 -> Product/2
  In/1 -> D linear3/1
  Sum6/1 -> on/off/1

== system P_decouple_cascade_rov/ ROV Dynamic   /pert1 ==
  In : Inport  Port=1  LatchInput=off
  inp : Inport  Port=2  LatchInput=off
  D linear3 : Gain  Gain=2  SaturateOnIntegerOverflow=on
  Product : Product  RndMeth=Zero
  Sine Wave-pert : Sin  Amplitude=0.1  SampleTime=0
  Sum6 : Sum  Inputs=|++  SaturateOnIntegerOverflow=on  InputSameDT=on
  on/off : Outport
  wires:
  D linear3/1 -> Sum6/1
  Sine Wave-pert/1 -> Product/1
  Product/1 -> Sum6/2
  inp/1 -> Product/2
  In/1 -> D linear3/1
  Sum6/1 -> on/off/1

== system P_decouple_cascade_rov/ ROV Dynamic   /pert2 ==
  In : Inport  Port=1  LatchInput=off
  inp : Inport  Port=2  LatchInput=off
  D linear3 : Gain  Gain=2  SaturateOnIntegerOverflow=on
  Product : Product  RndMeth=Zero
  Sine Wave-pert : Sin  Amplitude=0.1  SampleTime=0
  Sum6 : Sum  Inputs=|++  SaturateOnIntegerOverflow=on  InputSameDT=on
  on/off : Outport
  wires:
  D linear3/1 -> Sum6/1
  Sine Wave-pert/1 -> Product/1
  Product/1 -> Sum6/2
  inp/1 -> Product/2
  In/1 -> D linear3/1
  Sum6/1 -> on/off/1

== system P_decouple_cascade_rov/ ROV Dynamic   /upper limit (diag) ==
  In : Inport  Port=1  LatchInput=off
  inverse M : Gain  Gain=-diag([21.724-21.1403 51.7013-51.7012 94.3-92.451 4.2176-3.6191 7.1148-2.6427 4.7673-2.3033])  Multiplication=Matrix(K*u)  SaturateOnIntegerOverflow=on
  Out : Outport
  wires:
  inverse M/1 -> Out/1
  In/1 -> inverse M/1

== system P_decouple_cascade_rov/ ROV Dynamic   /upper limit (diag)    ==
  note: 7 8 9 10 11 12
  note: 1 2 3 4 5 6
  vel : Inport  Port=1  LatchInput=off
  (zg.W - zb.B)cY.sX : Fcn  Expr=-u[9]*u[3]*u[5]+u[8]*u[2]*u[6]
  (zg.W - zb.B)cY.sX1 : Fcn  Expr=u[9]*u[3]*u[4]-u[7]*u[1]*u[6]
  (zg.W - zb.B)cY.sX2 : Fcn  Expr=-u[8]*u[2]*u[4]+u[7]*u[1]*u[5]
  (zg.W - zb.B)cY.sX3 : Fcn  Expr=-u[9]*u[3]*u[2]+u[8]*u[2]*u[3]-u[12]*u[6]*u[5]+u[11]*u[5]*u[6]
  (zg.W - zb.B)cY.sX4 : Fcn  Expr=u[9]*u[3]*u[1]-u[7]*u[1]*u[3]+u[6]*u[12]*u[4]-u[4]*u[10]*u[6]
  (zg.W - zb.B)cY.sX5 : Fcn  Expr=-u[8]*u[2]*u[1]+u[7]*u[1]*u[2]-u[11]*u[5]*u[4]+u[10]*u[4]*u[5]
  Mux1 : Mux  Inputs=6
  Mux3 : Mux  Inputs=2
  Rg1 : Constant  Value="[MaU(1)  MaU(2)  MaU(3)  MaU(4)  MaU(5)  MaU(6) ]'"
  force : Outport
  wires:
  Mux1/1 -> force/1
  (zg.W - zb.B)cY.sX/1 -> Mux1/1
  (zg.W - zb.B)cY.sX1/1 -> Mux1/2
  (zg.W - zb.B)cY.sX2/1 -> Mux1/3
  (zg.W - zb.B)cY.sX3/1 -> Mux1/4
  (zg.W - zb.B)cY.sX4/1 -> Mux1/5
  (zg.W - zb.B)cY.sX5/1 -> Mux1/6
  vel/1 -> Mux3/1
  Rg1/1 -> Mux3/2
  Mux3/1 -> (zg.W - zb.B)cY.sX/1, (zg.W - zb.B)cY.sX1/1, (zg.W - zb.B)cY.sX4/1, (zg.W - zb.B)cY.sX5/1, (zg.W - zb.B)cY.sX3/1, (zg.W - zb.B)cY.sX2/1

== system P_decouple_cascade_rov/ ROV Dynamic   /upper limit (diag)   1 ==
  note: 7 8 9 10 11 12
  note: 1 2 3 4 5 6
  vel : Inport  Port=1  LatchInput=off
  (zg.W - zb.B)cY.sX : Fcn  Expr=-u[9]*u[3]*u[5]+u[8]*u[2]*u[6]
  (zg.W - zb.B)cY.sX1 : Fcn  Expr=u[9]*u[3]*u[4]-u[7]*u[1]*u[6]
  (zg.W - zb.B)cY.sX2 : Fcn  Expr=-u[8]*u[2]*u[4]+u[7]*u[1]*u[5]
  (zg.W - zb.B)cY.sX3 : Fcn  Expr=-u[9]*u[3]*u[2]+u[8]*u[2]*u[3]-u[12]*u[6]*u[5]+u[11]*u[5]*u[6]
  (zg.W - zb.B)cY.sX4 : Fcn  Expr=u[9]*u[3]*u[1]-u[7]*u[1]*u[3]+u[6]*u[12]*u[4]-u[4]*u[10]*u[6]
  (zg.W - zb.B)cY.sX5 : Fcn  Expr=-u[8]*u[2]*u[1]+u[7]*u[1]*u[2]-u[11]*u[5]*u[4]+u[10]*u[4]*u[5]
  Mux1 : Mux  Inputs=6
  Mux3 : Mux  Inputs=2
  Rg1 : Constant  Value="[Ma(1)  Ma(2)  Ma(3)  Ma(4)  Ma(5)  Ma(6) ]'"
  force : Outport
  wires:
  Mux1/1 -> force/1
  (zg.W - zb.B)cY.sX/1 -> Mux1/1
  (zg.W - zb.B)cY.sX1/1 -> Mux1/2
  (zg.W - zb.B)cY.sX2/1 -> Mux1/3
  (zg.W - zb.B)cY.sX3/1 -> Mux1/4
  (zg.W - zb.B)cY.sX4/1 -> Mux1/5
  (zg.W - zb.B)cY.sX5/1 -> Mux1/6
  vel/1 -> Mux3/1
  Rg1/1 -> Mux3/2
  Mux3/1 -> (zg.W - zb.B)cY.sX/1, (zg.W - zb.B)cY.sX1/1, (zg.W - zb.B)cY.sX4/1, (zg.W - zb.B)cY.sX5/1, (zg.W - zb.B)cY.sX3/1, (zg.W - zb.B)cY.sX2/1

== system P_decouple_cascade_rov/ ROV Dynamic   /upper limit1 ==
  In : Inport  Port=1  LatchInput=off
  inverse M : Gain  Gain=0  Multiplication=Matrix(K*u)  SaturateOnIntegerOverflow=on
  Out : Outport
  wires:
  inverse M/1 -> Out/1
  In/1 -> inverse M/1

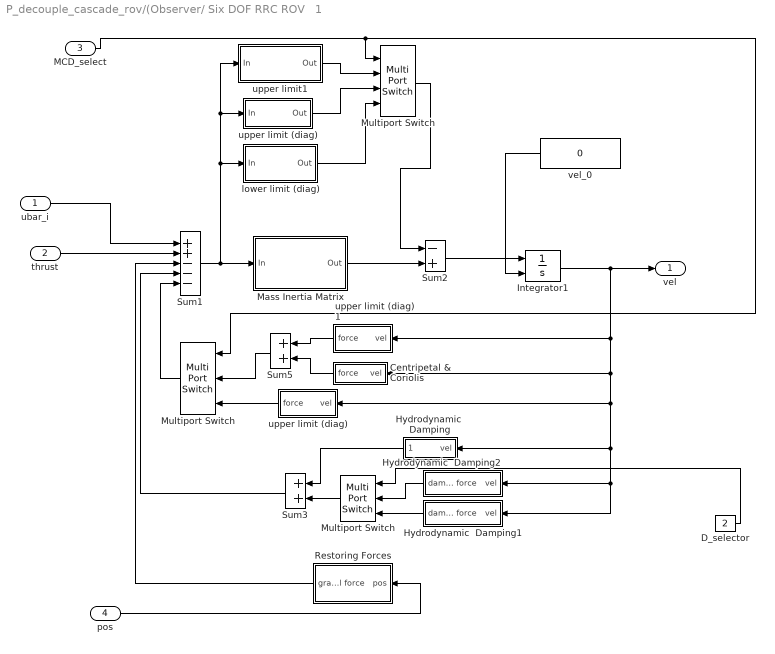
== system P_decouple_cascade_rov/(Observer/ Six DOF RRC ROV   1 ==
  ubar_i : Inport  Port=1  LatchInput=off
  "thrust " : Inport  Port=2  LatchInput=off
  MCD_select : Inport  Port=3  LatchInput=off
  "pos " : Inport  Port=4  LatchInput=off
  Centripetal & Coriolis : Subsystem  Orientation=left  AncestorBlock=rov_design_analysis/ROV Models/1. Six DOF RRC ROV II/Centripetal & Coriolis
      mask Display: disp('C')
  D_selector : Constant  Value=2
  Hydrodynamic  Damping : Subsystem  Orientation=left
      mask Display: disp('D')
  Hydrodynamic  Damping1 : Subsystem  Orientation=left
      mask Display: disp('perturb \nDamping')
  Hydrodynamic  Damping2 : Subsystem  Orientation=left
      mask Display: disp('Zero Perturb')
  Integrator1 : Integrator  InitialConditionSource=external
  Mass Inertia Matrix : Subsystem
      mask Display: disp('inv(MRB+MA)')
  Multiport Switch : MultiPortSwitch  Inputs=3
  "Multiport Switch  " : MultiPortSwitch  Orientation=left  Inputs=2
  "Multiport Switch    " : MultiPortSwitch  Orientation=left  Inputs=2
  Restoring Forces : Subsystem  Orientation=left
      mask Display: disp('Restoring\nForce')
  Sum1 : Sum  Inputs=++---  SaturateOnIntegerOverflow=on  InputSameDT=on
  Sum2 : Sum  Inputs=-+  SaturateOnIntegerOverflow=on  InputSameDT=on
  Sum3 : Sum  Orientation=left  SaturateOnIntegerOverflow=on  InputSameDT=on
  Sum5 : Sum  Orientation=left  SaturateOnIntegerOverflow=on  InputSameDT=on
  lower limit (diag) : Subsystem
      mask Display: disp('Perturb MA')
  upper limit (diag) : Subsystem
      mask Display: disp('Perturb MA')
  "upper limit (diag)   " : Subsystem  Orientation=left
      mask Display: disp('Perturb CA')
  upper limit (diag)   1 : Subsystem  Orientation=left
      mask Display: disp('CA')
  upper limit1 : Subsystem
      mask Display: disp('Zero Perturb')
  vel_0 : Constant  Orientation=left  Value=0  OutDataTypeMode=double
  vel : Outport
  wires:
  Restoring Forces/1(gravitational force) -> Sum1/3
  Sum1/1 -> Mass Inertia Matrix/1(In), upper limit1/1(In), upper limit (diag)/1(In), lower limit (diag)/1(In)
  "Multiport Switch  "/1 -> Sum1/5
  "pos "/1 -> Restoring Forces/1(pos)
  Mass Inertia Matrix/1(Out) -> Sum2/2
  upper limit1/1(Out) -> Multiport Switch/2
  upper limit (diag)/1(Out) -> Multiport Switch/3
  lower limit (diag)/1(Out) -> Multiport Switch/4
  Multiport Switch/1 -> Sum2/1
  "upper limit (diag)   "/1(force) -> "Multiport Switch  "/3
  Sum5/1 -> "Multiport Switch  "/2
  Hydrodynamic  Damping1/1(damping force) -> "Multiport Switch    "/3
  Hydrodynamic  Damping2/1(damping force) -> "Multiport Switch    "/2
  Sum3/1 -> Sum1/4
  "Multiport Switch    "/1 -> Sum3/2
  Hydrodynamic  Damping/1(damping force) -> Sum3/1
  MCD_select/1 -> Multiport Switch/1, "Multiport Switch  "/1
  upper limit (diag)   1/1(force) -> Sum5/1
  Centripetal & Coriolis/1(force) -> Sum5/2
  Sum2/1 -> Integrator1/1
  Integrator1/1 -> vel/1, upper limit (diag)   1/1(vel), Centripetal & Coriolis/1(vel), Hydrodynamic  Damping/1(vel), Hydrodynamic  Damping1/1(vel), Hydrodynamic  Damping2/1(vel), "upper limit (diag)   "/1(vel)
  ubar_i/1 -> Sum1/1
  vel_0/1 -> Integrator1/2
  D_selector/1 -> "Multiport Switch    "/1
  "thrust "/1 -> Sum1/2

== system P_decouple_cascade_rov/(Observer/Euler  Transformation1 ==
  vel : Inport  Port=1  LatchInput=off
  eta_0 : Inport  Port=2  LatchInput=off
  Demux : Demux  Outputs=2
  Demux1 : Demux  Outputs=2
  Intregrator2 : Integrator  InitialConditionSource=external
  Mux1 : Mux  Inputs=2
  Terminator : Terminator
  Transformation matrix R : Subsystem
      mask Display: disp('Transformation R')
  Transformation matrix T : Subsystem
      mask Display: disp('Transformation T')
  eout_hat : Outport  InitialOutput=0
  wires:
  Mux1/1 -> Intregrator2/1
  Intregrator2/1 -> eout_hat/1, Demux1/1
  Demux/2 -> Transformation matrix R/1(angular body  velocity)
  Demux/1 -> Transformation matrix T/1(translational body velocity)
  vel/1 -> Demux/1
  Demux1/2 -> Transformation matrix T/2(angular position), Transformation matrix R/2(angular position)
  Transformation matrix R/1(angular earth velocity) -> Mux1/2
  Transformation matrix T/1(translational earth velocity) -> Mux1/1
  Demux1/1 -> Terminator/1
  eta_0/1 -> Intregrator2/2

== system P_decouple_cascade_rov/(Observer/Thruster  Dynamic ==
  ubar_i : Inport  Port=1  LatchInput=off
  bout_err : Inport  Port=2  LatchInput=off
  Sum2 : Sum  Inputs=|++  OutDataTypeMode=double  SaturateOnIntegerOverflow=on
  Thruster configuration1 : Subsystem  AncestorBlock=|
      | rov_design_analysis/ROV Controller
      | Design
      | Applications/1. Heading autopilot/Thruster
      | configuration
      mask Display: disp('T')
  Thruster configuration4 : Subsystem  AncestorBlock=|
      | rov_design_analysis/ROV Controller
      | Design
      | Applications/1. Heading autopilot/Thruster
      | configuration
      mask Display: disp('T')
  thruster  dynamic     1 : Subsystem
  cont_out : Outport
  thruster_out : Outport  Port=2
  thruster_tot : Outport  Port=3
  wires:
  Thruster configuration1/1(output force) -> thruster_out/1
  Thruster configuration4/1(output force) -> cont_out/1
  thruster  dynamic     1/1(T) -> Thruster configuration1/1(input velocity), Sum2/2
  bout_err/1 -> thruster  dynamic     1/1(volt)
  ubar_i/1 -> Thruster configuration4/1(input velocity), Sum2/1
  Sum2/1 -> thruster_tot/1

== system P_decouple_cascade_rov/(Observer/inner-loop controller1 ==
  cont : Inport  Port=1  LatchInput=off
  err : Inport  Port=2  LatchInput=off
  M_select : Inport  Port=3  LatchInput=off
  Multiport Switch : MultiPortSwitch
  "inner -PI-decouple " : Subsystem
  inner -backstepping : Subsystem
  inner-P : Subsystem
  inner-sliding : Subsystem
  ubar_i : Outport
  wires:
  Multiport Switch/1 -> ubar_i/1
  cont/1 -> Multiport Switch/1
  "inner -PI-decouple "/1(" ") -> Multiport Switch/2
  inner-P/1(" ") -> Multiport Switch/3
  err/1 -> inner-P/1(P), inner-sliding/1(sliding), inner -backstepping/1(err), "inner -PI-decouple "/1(err)
  inner -backstepping/1(" ") -> Multiport Switch/4
  inner-sliding/1(" ") -> Multiport Switch/5
  M_select/1 -> inner -backstepping/2(M_select)

== system P_decouple_cascade_rov/Euler  Transformation/Transformation matrix R ==
  angular body  velocity : Inport  Port=1  LatchInput=off
  angular position : Inport  Port=2  LatchInput=off
  Mux : Mux  Inputs=3
  Row1 of T : Subsystem
      mask Display: disp('Row 1')
  Row2 of T : Subsystem
      mask Display: disp('Row 2')
  Row3 of T : Subsystem
      mask Display: disp('Row 3')
  angular earth velocity : Outport
  wires:
  angular position/1 -> Row3 of T/2(angular position), Row1 of T/2(angular position), Row2 of T/2(angular position)
  Mux/1 -> angular earth velocity/1
  Row3 of T/1(angular earth velocity (row 3)) -> Mux/3
  Row2 of T/1(angular earth velocity (row 2)) -> Mux/2
  Row1 of T/1(angular earth velocity (row 1)) -> Mux/1
  angular body  velocity/1 -> Row3 of T/1("angular body velocity "), Row2 of T/1("angular body velocity "), Row1 of T/1(angular body  velocity)

== system P_decouple_cascade_rov/Euler  Transformation/Transformation matrix T ==
  translational body velocity : Inport  Port=1  LatchInput=off
  angular position : Inport  Port=2  LatchInput=off
  Mux : Mux  Inputs=3
  Row1 of R : Subsystem
      mask Display: disp('Row 1')
  Row2 of R : Subsystem
      mask Display: disp('Row 2')
  Row3 of R : Subsystem
      mask Display: disp('Row 3')
  translational earth velocity : Outport  InitialOutput=0
  wires:
  Mux/1 -> translational earth velocity/1
  Row3 of R/1(translational earth velocity (row 3)) -> Mux/3
  Row2 of R/1(translational earth velocity (row 2)) -> Mux/2
  Row1 of R/1(translational earth velocity (row 1)) -> Mux/1
  angular position/1 -> Row3 of R/2(angular position), Row1 of R/2(angular position), Row2 of R/2(angular position)
  translational body velocity/1 -> Row1 of R/1(translational body velocity), Row2 of R/1(translational body velocity), Row3 of R/1(translational body velocity)

== system P_decouple_cascade_rov/Supervisor (Logic - based)/Mass Inertia Matrix1 ==
  In : Inport  Port=1  LatchInput=off
  inverse M : Gain  Gain=M-Ma  Multiplication=Matrix(K*u)  SaturateOnIntegerOverflow=on
  Out : Outport
  wires:
  inverse M/1 -> Out/1
  In/1 -> inverse M/1

== system P_decouple_cascade_rov/Supervisor (Logic - based)/Subsystem ==
  In : Inport  Port=1  LatchInput=off
  V : Inport  Port=2  LatchInput=off
  manual : Inport  Port=3  LatchInput=off
  Compare To Constant{,1..5} (6 alike) : simulink/Logic and Bit Operations/Compare To Constant  relop=>=  const=0  LogicOutDataTypeMode=uint8
  Demux : Demux  Outputs=6
  Mux : Mux  Inputs=6
  Product1 : Product  Inputs=3  RndMeth=Zero
  inner dwell : Outport
  wires:
  V/1 -> Demux/1
  Demux/1 -> Compare To Constant/1
  Demux/2 -> Compare To Constant1/1
  Demux/3 -> Compare To Constant2/1
  Demux/6 -> Compare To Constant5/1
  Demux/4 -> Compare To Constant3/1
  Demux/5 -> Compare To Constant4/1
  Compare To Constant/1 -> Mux/1
  Compare To Constant1/1 -> Mux/2
  Compare To Constant2/1 -> Mux/3
  Compare To Constant5/1 -> Mux/6
  Mux/1 -> Product1/2
  Compare To Constant3/1 -> Mux/4
  Compare To Constant4/1 -> Mux/5
  In/1 -> Product1/1
  Product1/1 -> inner dwell/1
  manual/1 -> Product1/3

== system P_decouple_cascade_rov/Supervisor (Logic - based)/Switching sequence ==
  Add2 : Sum  Inputs=+++++++  OutScaling=2^-10
  Signal Builder2 : Subsystem  Tag=STV Subsys  LoadFcn=sigbuilder_block('load');  StartFcn=sigbuilder_block('start');  StopFcn=sigbuilder_block('stop');  ClipboardFcn=sigbuilder_block('clipboard');  mask(Sigbuilder block){}
      mask help: Sigbuilder GUI
      mask init:
      | if ~strcmp(get_param(bdroot(gcbh),'SimulationStatus'),'stopped') tuvar = sigbuilder_block('maskInit'); end
      settings: CopyFcn=sigbuilder_block('copy');  DeleteFcn=sigbuilder_block('delete');  ModelCloseFcn=sigbuilder_block('modelClose');  PreSaveFcn=sigbuilder_block('preSave');  NameChangeFcn=sigbuilder_block('namechange');  OpenFcn=sigbuilder_block('open',[0 19.5 768 499.5 ]);  CloseFcn=sigbuilder_block('close');
      mask Display: plot(0,0,100,100,[10,10,40,40,10],[80,20,20,80,80],[40,10],[50,50], [40,27,10],[65,72,56],[40,25,25,10],[28,28,43,43]);
  " " : Outport
  wires:
  Add2/1 -> " "/1
  Signal Builder2/7(Signal 7) -> Add2/7
  Signal Builder2/6(Signal 6) -> Add2/6
  Signal Builder2/5(Signal 5) -> Add2/5
  Signal Builder2/4(Signal 4) -> Add2/4
  Signal Builder2/3(Signal 3) -> Add2/3
  Signal Builder2/2(Signal 2) -> Add2/2
  Signal Builder2/1(Signal 1) -> Add2/1

== system P_decouple_cascade_rov/Supervisor (Logic - based)/Switching sequence1 ==
  Add2 : Sum  Inputs=+++++++  OutScaling=2^-10
  Signal Builder2 : Subsystem  Tag=STV Subsys  LoadFcn=sigbuilder_block('load');  StartFcn=sigbuilder_block('start');  StopFcn=sigbuilder_block('stop');  ClipboardFcn=sigbuilder_block('clipboard');  mask(Sigbuilder block){}
      mask help: Sigbuilder GUI
      mask init:
      | if ~strcmp(get_param(bdroot(gcbh),'SimulationStatus'),'stopped') tuvar = sigbuilder_block('maskInit'); end
      settings: CopyFcn=sigbuilder_block('copy');  DeleteFcn=sigbuilder_block('delete');  ModelCloseFcn=sigbuilder_block('modelClose');  PreSaveFcn=sigbuilder_block('preSave');  NameChangeFcn=sigbuilder_block('namechange');  OpenFcn=sigbuilder_block('open',[0 19.5 768 499.5 ]);  CloseFcn=sigbuilder_block('close');
      mask Display: plot(0,0,100,100,[10,10,40,40,10],[80,20,20,80,80],[40,10],[50,50], [40,27,10],[65,72,56],[40,25,25,10],[28,28,43,43]);
  " " : Outport
  wires:
  Add2/1 -> " "/1
  Signal Builder2/7(Signal 7) -> Add2/7
  Signal Builder2/6(Signal 6) -> Add2/6
  Signal Builder2/5(Signal 5) -> Add2/5
  Signal Builder2/4(Signal 4) -> Add2/4
  Signal Builder2/3(Signal 3) -> Add2/3
  Signal Builder2/2(Signal 2) -> Add2/2
  Signal Builder2/1(Signal 1) -> Add2/1

== system P_decouple_cascade_rov/Thruster  Dynamic/Thruster configuration1 ==
  input velocity : Inport  Orientation=up  Port=1  LatchInput=off
  Thruster Matrix : Gain  Gain=T  Multiplication=Matrix(K*u)  SaturateOnIntegerOverflow=on
  output force : Outport  InitialOutput=0
  wires:
  input velocity/1 -> Thruster Matrix/1
  Thruster Matrix/1 -> output force/1

== system P_decouple_cascade_rov/Thruster  Dynamic/Thruster configuration4 ==
  input velocity : Inport  Orientation=up  Port=1  LatchInput=off
  Thruster Matrix : Gain  Gain=T  Multiplication=Matrix(K*u)  SaturateOnIntegerOverflow=on
  output force : Outport  InitialOutput=0
  wires:
  input velocity/1 -> Thruster Matrix/1
  Thruster Matrix/1 -> output force/1

== system P_decouple_cascade_rov/Thruster  Dynamic/thruster  dynamic     1 ==
  volt : Inport  Orientation=down  Port=1  LatchInput=off
  Gain2 : Gain  Gain=0.5  SaturateOnIntegerOverflow=on
  Saturation : Saturate  UpperLimit=70  LowerLimit=-70
  "thruster  alloc. " : Subsystem
  T : Outport
  wires:
  volt/1 -> "thruster  alloc. "/1(err)
  "thruster  alloc. "/1(u) -> Gain2/1
  Saturation/1 -> T/1
  Gain2/1 -> Saturation/1

== system P_decouple_cascade_rov/inner-loop controller/inner -PI-decouple  ==
  err : Inport  Port=1  LatchInput=off
  Centripetal & Coriolis : Subsystem  AncestorBlock=rov_design_analysis/ROV Models/1. Six DOF RRC ROV II/Centripetal & Coriolis
      mask Display: disp('C')
  Gain2 : Gain  SaturateOnIntegerOverflow=on
  Hydrodynamic  Damping : Subsystem
      mask Display: disp('D')
  Hydrodynamic  Damping1 : Subsystem
      mask Display: disp('Perturb D')
  Sum : Sum  Inputs=|-++  SaturateOnIntegerOverflow=on  InputSameDT=on
  Sum1 : Sum  Inputs=+++  SaturateOnIntegerOverflow=on  InputSameDT=on
  Sum5 : Sum  Inputs=|++  SaturateOnIntegerOverflow=on  InputSameDT=on
  inner-PI : Subsystem
  thruster  dynamic     1 : Subsystem
  "upper limit (diag)   " : Subsystem
      mask Display: disp('Perturb CA')
  upper limit (diag)   1 : Subsystem
      mask Display: disp('CA')
  " " : Outport
  wires:
  err/1 -> upper limit (diag)   1/1(vel), Centripetal & Coriolis/1(vel), "upper limit (diag)   "/1(vel), Hydrodynamic  Damping/1(vel), Hydrodynamic  Damping1/1(vel), inner-PI/1(PI)
  upper limit (diag)   1/1(force) -> Sum1/1
  Centripetal & Coriolis/1(force) -> Sum1/2
  Hydrodynamic  Damping1/1(damping force) -> Sum5/2
  inner-PI/1(" ") -> Gain2/1
  "upper limit (diag)   "/1(force) -> Sum1/3
  Hydrodynamic  Damping/1(damping force) -> Sum5/1
  Gain2/1 -> Sum/1
  Sum5/1 -> Sum/3
  Sum1/1 -> Sum/2
  Sum/1 -> thruster  dynamic     1/1(volt)
  thruster  dynamic     1/1(T) -> " "/1
